simulink model "whirleybird_animation"  (Simulink 8.3)
settings: Solver=ode45  StartTime=0.0  StopTime=inf  RelTol=1e-3
undefined symbols (not defined in the file or in its folder): drawWhirleybird
libraries: simulink x3
settings Model: Creator=beard  LastModifiedBy=jhl48
settings OptimizationCC: ExpressionDepthLimit=2147483647  InitFltsAndDblsToZero=on
settings DebuggingCC: FcnCallInpInsideContextMsg=UseLocalSettings

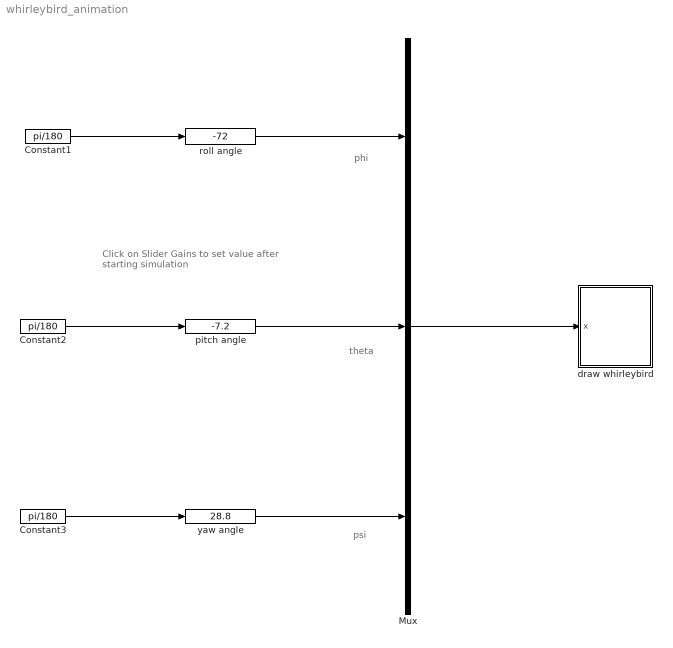
== system whirleybird_animation ==
  note: phi
  note: theta
  note: psi
  note: Click on Slider Gains to set value
      | after starting simulation
  Constant1 : Constant  Value=pi/180
  Constant2 : Constant  Value=pi/180
  Constant3 : Constant  Value=pi/180
  Mux : Mux  Inputs=3
  draw whirleybird : Subsystem
      mask Display: image(imread('tv.jpg'))
  pitch angle : simulink/Math Operations/Slider Gain  low=-180  gain=-7.2  high=180
  roll angle : simulink/Math Operations/Slider Gain  low=-180  gain=-72  high=180
  "yaw angle " : simulink/Math Operations/Slider Gain  low=-180  gain=28.8  high=180
  wires:
  Mux/1 -> draw whirleybird/1(x)
  roll angle/1 -> Mux/1
  Constant1/1 -> roll angle/1
  pitch angle/1 -> Mux/2
  Constant2/1 -> pitch angle/1
  "yaw angle "/1 -> Mux/3
  Constant3/1 -> "yaw angle "/1

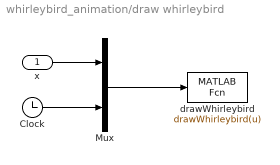
== system whirleybird_animation/draw whirleybird ==
  x : Inport
  Clock : Clock
  Mux : Mux  Inputs=2
  drawWhirleybird : MATLABFcn  MATLABFcn=drawWhirleybird(u)  OutputDimensions=0  SampleTime=0.1
  wires:
  Mux/1 -> drawWhirleybird/1
  x/1 -> Mux/1
  Clock/1 -> Mux/2
